simulink model "SS1"  (R2020a)
settings: Solver=VariableStepAuto  StartTime=0.0  StopTime=10.0  RelTol=1e-3
settings Model: Creator=Asus  LastModifiedBy=Asus

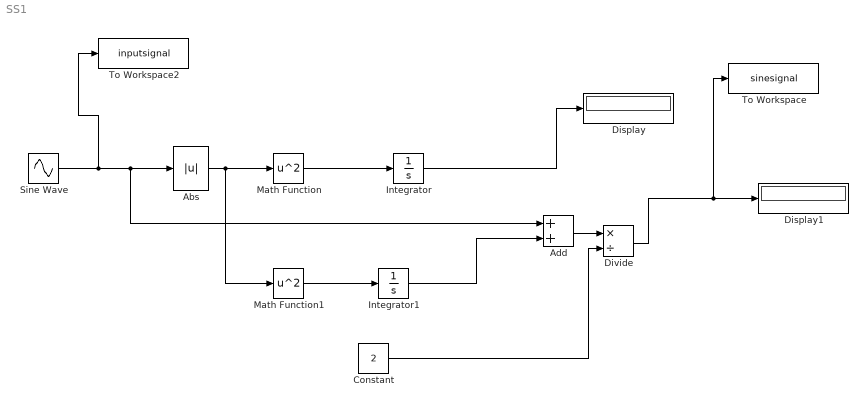
== system SS1 ==
  Abs : Abs
  Add : Sum
  Constant : Constant  Value=2
  Display : Display
  Display1 : Display
  Divide : Product  Inputs=*/
  Integrator : Integrator  LimitOutput=on
  Integrator1 : Integrator  LimitOutput=on
  Math Function : Math  Operator=square  SaturateOnIntegerOverflow=on
  Math Function1 : Math  Operator=square  SaturateOnIntegerOverflow=on
  Sine Wave : Sin  SampleTime=0
  To Workspace : ToWorkspace  VariableName=sinesignal  SaveFormat=Timeseries  SampleTime=-1
  To Workspace2 : ToWorkspace  VariableName=inputsignal  SaveFormat=Timeseries  SampleTime=-1
  wires:
  Math Function/1 -> Integrator/1
  Math Function1/1 -> Integrator1/1
  Integrator1/1 -> Add/2
  Constant/1 -> Divide/2
  Abs/1 -> Math Function1/1, Math Function/1
  Sine Wave/1 -> To Workspace2/1, Add/1, Abs/1
  Integrator/1 -> Display/1
  Divide/1 -> To Workspace/1, Display1/1
  Add/1 -> Divide/1
